simulink model "LowPass_Test"  (R2022b)
settings: Solver=FixedStepAuto  StartTime=0.0  StopTime=1  FixedStep=1e-4  MaxStep=1e-3  RelTol=1e-3
libraries: cstblocks x1
settings Model: Creator=Rio  LastModifiedBy=Rio

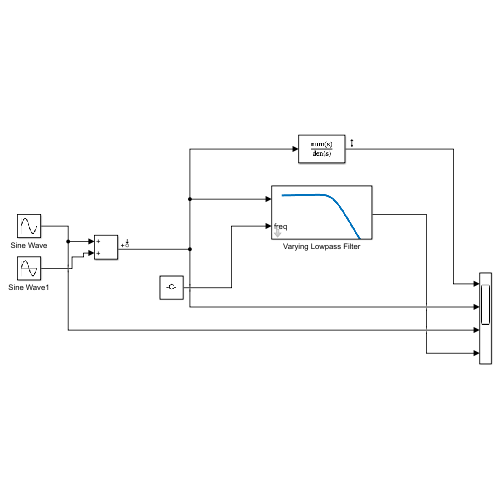
[thumbnail: Simulink's stored preview of the top-level diagram]
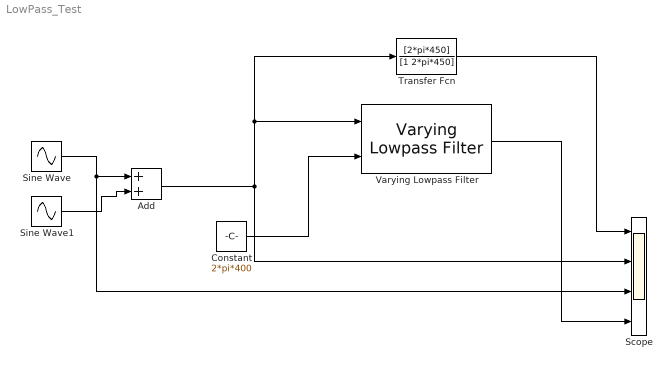
== system LowPass_Test ==
  Add : Sum
  Constant : Constant  Value=2*pi*400
  Scope : Scope  NumInputPorts=4
  Sine Wave : Sin  Frequency=2*pi*300  SampleTime=0
  Sine Wave1 : Sin  Amplitude=0.5  Frequency=2*pi*1000  SampleTime=0
  Transfer Fcn : TransferFcn  Numerator=[2*pi*450]  Denominator=[1 2*pi*450]
  Varying Lowpass Filter : cstblocks/Linear Parameter Varying/Varying Lowpass Filter  N=4
  wires:
  Sine Wave1/1 -> Add/2
  Add/1 -> Scope/2, Transfer Fcn/1, Varying Lowpass Filter/1
  Constant/1 -> Varying Lowpass Filter/2
  Sine Wave/1 -> Scope/3, Add/1
  Varying Lowpass Filter/1 -> Scope/4
  Transfer Fcn/1 -> Scope/1
